simulink model "tasks500Hz"  (R2014a)
settings: Solver=FixedStepDiscrete  StartTime=0.0  StopTime=simTime  FixedStep=controlDT  RelTol=1e-3
values from neighbouring files (symbols this model uses):
  controlDT = 1 / 500    (= 0.002)    [setup.m]
  eepromConfig = p    [setup.m]
  triYawRateDenLP = p    [setup.m]
  triYawRateNumLP = p    [setup.m]
undefined symbols (not defined in the file or in its folder): DiscIntNeverNeededParam, mixHexX, mixQuadX, mixTri, mixY6
libraries: simulink x9, mahoneyAHRSlibrary x1
settings Model: Creator=John Ihlein  LastModifiedBy=John Ihlein
settings DataIOCC: SaveFormat=Structure  SaveOutput=off  SaveTime=off
settings OptimizationCC: InlineParams=on  DefaultUnderspecifiedDataType=single  InlineInvariantSignals=on  PassReuseOutputArgsAs=Individual arguments  StateBitsets=on  DataBitsets=on  ZeroExternalMemoryAtStartup=off  ZeroInternalMemoryAtStartup=off  EfficientFloat2IntCast=on  OptimizeModelRefInitCode=on  LifeSpan=1
settings DebuggingCC: ParameterPrecisionLossMsg=none  UniqueDataStoreMsg=error  AssertControl=DisableAll
settings HardwareCC: ProdLargestAtomicInteger=Integer  ProdLargestAtomicFloat=Float  ProdIntDivRoundTo=Zero  ProdEndianess=LittleEndian  ProdHWDeviceType=STMicroelectronics->STM32F4xx 32-bit Cortex-M4
settings RTWCC: SystemTargetFile=ert.tlc  GenCodeOnly=on  TemplateMakefile=ert_default_tmf  Description=Embedded Coder  ProcessScript=ert_make_rtw_hook
settings CodeAppCC: IgnoreCustomStorageClasses=off  IgnoreTestpoints=on
settings ERTTargetCC: ParMdlRefBuildCompliant=on  CompOptLevelCompliant=on  ConcurrentExecutionCompliant=on  IncludeMdlTerminateFcn=off  ERTFirstTimeCompliant=on  SupportNonFinite=off  ParenthesesLevel=Maximum  ModelStepFunctionPrototypeControlCompliant=on  CPPClassGenCompliant=on  InlinedParameterPlacement=Hierarchical  ERTCustomFileTemplate=example_file_process.tlc  ERTFilePackagingFormat=Compact

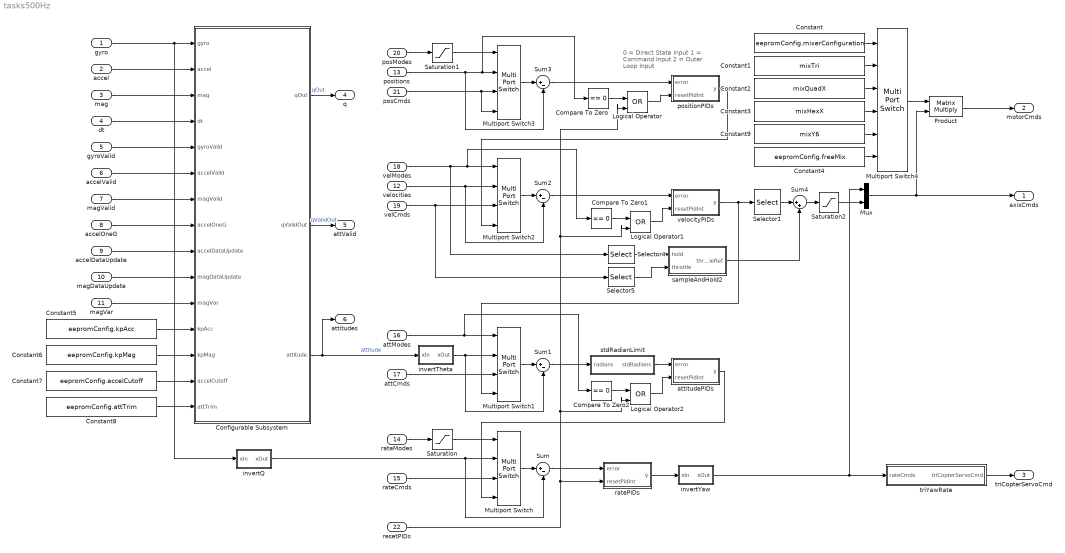
== system tasks500Hz ==
  note: 0 = Direct State Input
      | 1 = Command Input
      | 2 = Outer Loop Input
  "gyro " : Inport  OutDataTypeStr=single  PortDimensions=3  SampleTime=controlDT
  accel : Inport  Port=2  OutDataTypeStr=single  PortDimensions=3  SampleTime=controlDT
  mag : Inport  Port=3  OutDataTypeStr=single  PortDimensions=3  SampleTime=controlDT
  dt : Inport  Port=4  OutDataTypeStr=single  PortDimensions=1  SampleTime=controlDT
  gyroValid : Inport  Port=5  OutDataTypeStr=uint8  PortDimensions=1  SampleTime=controlDT
  accelValid : Inport  Port=6  OutDataTypeStr=uint8  PortDimensions=1  SampleTime=controlDT
  magValid : Inport  Port=7  OutDataTypeStr=uint8  PortDimensions=1  SampleTime=controlDT
  accelOneG : Inport  Port=8  OutDataTypeStr=single  PortDimensions=1  SampleTime=controlDT
  accelDataUpdate : Inport  Port=9  OutDataTypeStr=uint8  PortDimensions=1  SampleTime=controlDT
  magDataUpdate : Inport  Port=10  OutDataTypeStr=uint8  PortDimensions=1  SampleTime=controlDT
  magVar : Inport  Port=11  OutDataTypeStr=single  PortDimensions=1  SampleTime=controlDT
  velocities : Inport  Port=12  OutDataTypeStr=single  PortDimensions=3  SampleTime=controlDT
  positions : Inport  Port=13  OutDataTypeStr=single  PortDimensions=3  SampleTime=controlDT
  rateModes : Inport  Port=14  OutDataTypeStr=uint8  PortDimensions=3  SampleTime=controlDT
  rateCmds : Inport  Port=15  OutDataTypeStr=single  PortDimensions=3  SampleTime=controlDT
  attModes : Inport  Port=16  OutDataTypeStr=uint8  PortDimensions=3  SampleTime=controlDT
  attCmds : Inport  Port=17  OutDataTypeStr=single  PortDimensions=3  SampleTime=controlDT
  velModes : Inport  Port=18  OutDataTypeStr=uint8  PortDimensions=3  SampleTime=controlDT
  velCmds : Inport  Port=19  OutDataTypeStr=single  PortDimensions=3  SampleTime=controlDT
  posModes : Inport  Port=20  OutDataTypeStr=uint8  PortDimensions=3  SampleTime=controlDT
  posCmds : Inport  Port=21  OutDataTypeStr=single  PortDimensions=3  SampleTime=controlDT
  resetPIDs : Inport  Port=22  OutDataTypeStr=uint8  PortDimensions=1  SampleTime=controlDT
  Compare To Zero : simulink/Logic and Bit Operations/Compare To Zero  relop===  OutDataTypeStr=boolean
  Compare To Zero1 : simulink/Logic and Bit Operations/Compare To Zero  relop===  OutDataTypeStr=boolean
  Compare To Zero2 : simulink/Logic and Bit Operations/Compare To Zero  relop===  OutDataTypeStr=boolean
  Configurable Subsystem : Subsystem  BlockChoice=mahonyAHRS_MC
      settings: AttributesFormatString=%<BlockChoice>  MemberBlocks=mahonyAHRS_MC,mahonyAHRS_SL
      settings: TemplateBlock=|
      | mahoneyAHRSlibrary/Configurable
      | Subsystem
  Constant : Constant  Value=eepromConfig.mixerConfiguration  OutDataTypeStr=single  SampleTime=controlDT
  Constant1 : Constant  Value=mixTri  OutDataTypeStr=single  SampleTime=controlDT
  Constant2 : Constant  Value=mixQuadX  OutDataTypeStr=single  SampleTime=controlDT
  Constant3 : Constant  Value=mixHexX  OutDataTypeStr=single  SampleTime=controlDT
  Constant4 : Constant  Value=eepromConfig.freeMix  OutDataTypeStr=single  SampleTime=controlDT
  Constant5 : Constant  Value=eepromConfig.kpAcc  OutDataTypeStr=single  SampleTime=controlDT
  Constant6 : Constant  Value=eepromConfig.kpMag  OutDataTypeStr=single  SampleTime=controlDT
  Constant7 : Constant  Value=eepromConfig.accelCutoff  OutDataTypeStr=single  SampleTime=controlDT
  Constant8 : Constant  Value=eepromConfig.attTrim  OutDataTypeStr=single  SampleTime=controlDT
  Constant9 : Constant  Value=mixY6  OutDataTypeStr=single  SampleTime=controlDT
  Logical Operator : Logic  Operator=OR  IconShape=distinctive  AllPortsSameDT=off  OutDataTypeStr=boolean
  Logical Operator1 : Logic  Operator=OR  IconShape=distinctive  AllPortsSameDT=off  OutDataTypeStr=boolean
  Logical Operator2 : Logic  Operator=OR  IconShape=distinctive  AllPortsSameDT=off  OutDataTypeStr=boolean
  Multiport Switch4 : MultiPortSwitch  DataPortOrder=Zero-based contiguous  Inputs=5
  Multiport Switch{,1..3} (4 alike) : MultiPortSwitch  DataPortOrder=Zero-based contiguous
  Mux : Mux  Inputs=2
  Product : Product  Multiplication=Matrix(*)
  Saturation : Saturate  UpperLimit=2  LowerLimit=1
  Saturation1 : Saturate  UpperLimit=1  LowerLimit=0
  Saturation2 : Saturate  UpperLimit=4000  LowerLimit=2000
  Selector1 : Selector  IndexMode=Zero-based  InputPortWidth=3  Indices=[2]
  Selector4 : Selector  IndexMode=Zero-based  InputPortWidth=3  Indices=[2]
  Selector5 : Selector  IndexMode=Zero-based  InputPortWidth=3  Indices=[2]
  Sum{,1..3} (4 alike) : Sum  Inputs=|+-
  Sum4 : Sum  Inputs=|++
  attitudePIDs : Subsystem  mask{P=eepromConfig.attitudeP, I=eepromConfig.attitudeI, D=eepromConfig.attitudeD, N=100, Kb=100, pidLimit=eepromConfig.attitudeLimit}
      mask prompts: P "PID P Gain"; I "PID I Gain"; D "PID D Gain"; N "PID N"; Kb "PID Kb"; pidLimit "PID Limit"
  invertQ : Subsystem
  invertTheta : Subsystem
  invertYaw : Subsystem
  positionPIDs : Subsystem  mask{P=eepromConfig.positionP, I=eepromConfig.positionI, D=eepromConfig.positionD, N=100, Kb=100, pidLimit=eepromConfig.positionLimit}
      mask prompts: P "PID P Gain"; I "PID I Gain"; D "PID D Gain"; N "PID N"; Kb "PID Kb"; pidLimit "PID Limit"
  ratePIDs : Subsystem  mask{P=eepromConfig.rateP, I=eepromConfig.rateI, D=eepromConfig.rateD, N=100, Kb=100, pidLimit=eepromConfig.rateLimit}
      mask prompts: P "PID P Gain"; I "PID I Gain"; D "PID D Gain"; N "PID N"; Kb "PID Kb"; pidLimit "PID Limit"
  sampleAndHold2 : Subsystem
  stdRadianLimit : Subsystem
  triYawRate : Subsystem
  velocityPIDs : Subsystem  mask{P=eepromConfig.velocityP, I=eepromConfig.velocityI, D=eepromConfig.velocityD, N=100, Kb=100, pidLimit=eepromConfig.velocityLimit}
      mask prompts: P "PID P Gain"; I "PID I Gain"; D "PID D Gain"; N "PID N"; Kb "PID Kb"; pidLimit "PID Limit"
  axisCmds : Outport  OutDataTypeStr=single  PortDimensions=4  SampleTime=controlDT
  motorCmds : Outport  Port=2  OutDataTypeStr=single  PortDimensions=numMotors  SampleTime=controlDT
  triCopterServoCmd : Outport  Port=3  OutDataTypeStr=single  PortDimensions=1  SampleTime=controlDT
  q : Outport  Port=4  OutDataTypeStr=single  PortDimensions=[1 4]  SampleTime=controlDT
  attValid : Outport  Port=5  OutDataTypeStr=uint8  PortDimensions=1  SampleTime=controlDT
  attitudes : Outport  Port=6  OutDataTypeStr=single  PortDimensions=3  SampleTime=controlDT
  wires:
  attModes/1 -> Multiport Switch1/1, Compare To Zero2/1
  Sum1/1 -> stdRadianLimit/1(radians)
  velCmds/1 -> Multiport Switch2/3, Selector5/1
  velModes/1 -> Multiport Switch2/1, Compare To Zero1/1, Selector4/1
  Multiport Switch3/1 -> Sum3/1
  stdRadianLimit/1(stdRadians) -> attitudePIDs/1(error)
  attCmds/1 -> Multiport Switch1/3
  Multiport Switch/1 -> Sum/1
  Selector1/1 -> Sum4/1
  Multiport Switch2/1 -> Sum2/1
  velocityPIDs/1(y) -> Multiport Switch1/4, Selector1/1
  Sum3/1 -> positionPIDs/1(error)
  positions/1 -> Multiport Switch3/2, Compare To Zero/1, Sum3/2
  Multiport Switch1/1 -> Sum1/1
  Saturation/1 -> Multiport Switch/1
  sampleAndHold2/1(throttleRef) -> Sum4/2
  Selector4/1 -> sampleAndHold2/1(hold)
  Selector5/1 -> sampleAndHold2/2(throttle)
  rateModes/1 -> Saturation/1
  attitudePIDs/1(y) -> Multiport Switch/4
  posCmds/1 -> Multiport Switch3/3, Multiport Switch3/4
  rateCmds/1 -> Multiport Switch/3
  resetPIDs/1 -> Logical Operator/2, Logical Operator1/2, Logical Operator2/2, ratePIDs/2(resetPidInt)
  Sum/1 -> ratePIDs/1(error)
  velocities/1 -> Multiport Switch2/2, Sum2/2
  positionPIDs/1(y) -> Multiport Switch2/4
  Saturation1/1 -> Multiport Switch3/1
  posModes/1 -> Saturation1/1
  Mux/1 -> axisCmds/1, Product/2
  Sum4/1 -> Saturation2/1
  ratePIDs/1(y) -> invertYaw/1(xIn)
  Compare To Zero/1 -> Logical Operator/1
  Logical Operator/1 -> positionPIDs/2(resetPidInt)
  Compare To Zero1/1 -> Logical Operator1/1
  Logical Operator1/1 -> velocityPIDs/2(resetPidInt)
  Logical Operator2/1 -> attitudePIDs/2(resetPidInt)
  Compare To Zero2/1 -> Logical Operator2/1
  invertQ/1(xOut) -> Multiport Switch/2, Sum/2
  invertTheta/1(xOut) -> Multiport Switch1/2, Sum1/2
  Saturation2/1 -> Mux/2
  Constant/1 -> Multiport Switch4/1
  Constant1/1 -> Multiport Switch4/2
  Constant2/1 -> Multiport Switch4/3
  Constant3/1 -> Multiport Switch4/4
  Multiport Switch4/1 -> Product/1
  Product/1 -> motorCmds/1
  invertYaw/1(xOut) -> Mux/1, triYawRate/1(rateCmds)
  triYawRate/1(triCopterServoCmd) -> triCopterServoCmd/1
  Sum2/1 -> velocityPIDs/1(error)
  Configurable Subsystem/3(attitude) -> attitudes/1, invertTheta/1(xIn)  "attitude"
  Configurable Subsystem/2(qValidOut) -> attValid/1  "qValidOut"
  magDataUpdate/1 -> Configurable Subsystem/10(magDataUpdate)
  accel/1 -> Configurable Subsystem/2(accel)
  mag/1 -> Configurable Subsystem/3(mag)
  magValid/1 -> Configurable Subsystem/7(magValid)
  accelValid/1 -> Configurable Subsystem/6(accelValid)
  gyroValid/1 -> Configurable Subsystem/5(gyroValid)
  "gyro "/1 -> Configurable Subsystem/1(gyro), invertQ/1(xIn)
  Configurable Subsystem/1(qOut) -> q/1  "qOut"
  accelDataUpdate/1 -> Configurable Subsystem/9(accelDataUpdate)
  magVar/1 -> Configurable Subsystem/11(magVar)
  Constant5/1 -> Configurable Subsystem/12(kpAcc)
  Constant6/1 -> Configurable Subsystem/13(kpMag)
  Constant7/1 -> Configurable Subsystem/14(accelCutoff)
  Constant8/1 -> Configurable Subsystem/15(attTrim)
  dt/1 -> Configurable Subsystem/4(dt)
  accelOneG/1 -> Configurable Subsystem/8(accelOneG)
  Constant4/1 -> Multiport Switch4/6
  Constant9/1 -> Multiport Switch4/5

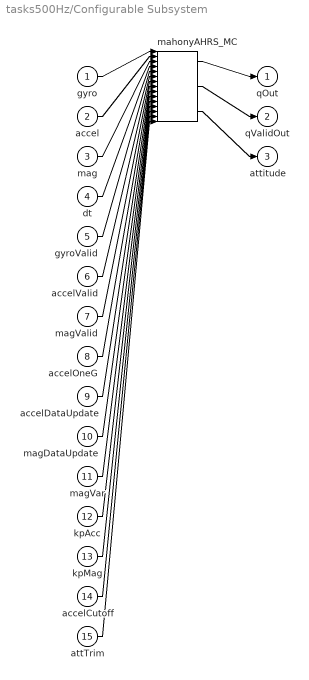
== system tasks500Hz/Configurable Subsystem ==
  gyro : Inport
  accel : Inport  Port=2
  mag : Inport  Port=3
  dt : Inport  Port=4
  gyroValid : Inport  Port=5
  accelValid : Inport  Port=6
  magValid : Inport  Port=7
  accelOneG : Inport  Port=8
  accelDataUpdate : Inport  Port=9
  magDataUpdate : Inport  Port=10
  magVar : Inport  Port=11
  kpAcc : Inport  Port=12
  kpMag : Inport  Port=13
  accelCutoff : Inport  Port=14
  attTrim : Inport  Port=15
  mahonyAHRS_MC : mahoneyAHRSlibrary/mahonyAHRS_MC
  qOut : Outport
  qValidOut : Outport  Port=2
  attitude : Outport  Port=3
  wires:
  gyro/1 -> mahonyAHRS_MC/1
  accel/1 -> mahonyAHRS_MC/2
  mag/1 -> mahonyAHRS_MC/3
  dt/1 -> mahonyAHRS_MC/4
  gyroValid/1 -> mahonyAHRS_MC/5
  accelValid/1 -> mahonyAHRS_MC/6
  magValid/1 -> mahonyAHRS_MC/7
  accelOneG/1 -> mahonyAHRS_MC/8
  accelDataUpdate/1 -> mahonyAHRS_MC/9
  magDataUpdate/1 -> mahonyAHRS_MC/10
  magVar/1 -> mahonyAHRS_MC/11
  kpAcc/1 -> mahonyAHRS_MC/12
  kpMag/1 -> mahonyAHRS_MC/13
  accelCutoff/1 -> mahonyAHRS_MC/14
  attTrim/1 -> mahonyAHRS_MC/15
  mahonyAHRS_MC/1 -> qOut/1
  mahonyAHRS_MC/2 -> qValidOut/1
  mahonyAHRS_MC/3 -> attitude/1

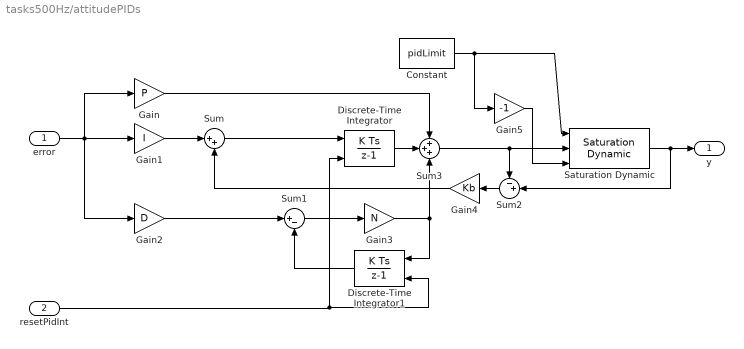
== system tasks500Hz/attitudePIDs ==
  error : Inport
  resetPidInt : Inport  Port=2
  Constant : Constant  Value=pidLimit
  Discrete-Time Integrator : DiscreteIntegrator  ExternalReset=level  SampleTime=-1  ICPrevOutput=DiscIntNeverNeededParam  ICPrevScaledInput=DiscIntNeverNeededParam
  Discrete-Time Integrator1 : DiscreteIntegrator  ExternalReset=level  SampleTime=-1  ICPrevOutput=DiscIntNeverNeededParam  ICPrevScaledInput=DiscIntNeverNeededParam
  Gain : Gain  Gain=P
  Gain1 : Gain  Gain=I
  Gain2 : Gain  Gain=D
  Gain3 : Gain  Gain=N
  Gain4 : Gain  Gain=Kb
  Gain5 : Gain  Gain=-1
  Saturation Dynamic : simulink/Discontinuities/Saturation Dynamic  OutMin=[]  OutMax=[]  OutDataTypeStr=Inherit: Same as second input  OutDataType=fixdt(1, 16)  OutScaling=2^-10  DoSatur=off
  Sum : Sum  Inputs=|++
  Sum1 : Sum  Inputs=|+-
  Sum2 : Sum  Inputs=-+|
  Sum3 : Sum  Inputs=+++
  y : Outport
  wires:
  Constant/1 -> Saturation Dynamic/1, Gain5/1
  Gain5/1 -> Saturation Dynamic/3
  Gain/1 -> Sum3/1
  error/1 -> Gain1/1, Gain2/1, Gain/1
  Saturation Dynamic/1 -> Sum2/2, y/1
  Discrete-Time Integrator1/1 -> Sum1/2
  Sum2/1 -> Gain4/1
  Discrete-Time Integrator/1 -> Sum3/2
  Gain2/1 -> Sum1/1
  Gain3/1 -> Sum3/3, Discrete-Time Integrator1/1
  Sum/1 -> Discrete-Time Integrator/1
  Gain1/1 -> Sum/1
  Sum3/1 -> Sum2/1, Saturation Dynamic/2
  Sum1/1 -> Gain3/1
  Gain4/1 -> Sum/2
  resetPidInt/1 -> Discrete-Time Integrator/2, Discrete-Time Integrator1/2

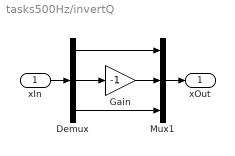
== system tasks500Hz/invertQ ==
  xIn : Inport
  Demux : Demux  Outputs=3
  Gain : Gain  Gain=-1
  Mux1 : Mux  Inputs=3
  xOut : Outport
  wires:
  Gain/1 -> Mux1/2
  Demux/3 -> Mux1/3
  Demux/1 -> Mux1/1
  Mux1/1 -> xOut/1
  Demux/2 -> Gain/1
  xIn/1 -> Demux/1

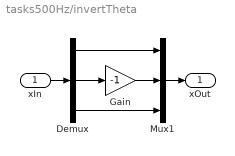
== system tasks500Hz/invertTheta ==
  xIn : Inport
  Demux : Demux  Outputs=3
  Gain : Gain  Gain=-1
  Mux1 : Mux  Inputs=3
  xOut : Outport
  wires:
  Demux/3 -> Mux1/3
  Demux/1 -> Mux1/1
  xIn/1 -> Demux/1
  Demux/2 -> Gain/1
  Mux1/1 -> xOut/1
  Gain/1 -> Mux1/2

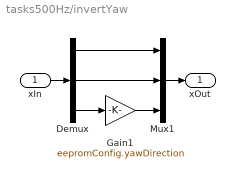
== system tasks500Hz/invertYaw ==
  xIn : Inport
  Demux : Demux  Outputs=3
  Gain1 : Gain  Gain=eepromConfig.yawDirection
  Mux1 : Mux  Inputs=3
  xOut : Outport
  wires:
  Gain1/1 -> Mux1/3
  Demux/2 -> Mux1/2
  Mux1/1 -> xOut/1
  xIn/1 -> Demux/1
  Demux/1 -> Mux1/1
  Demux/3 -> Gain1/1

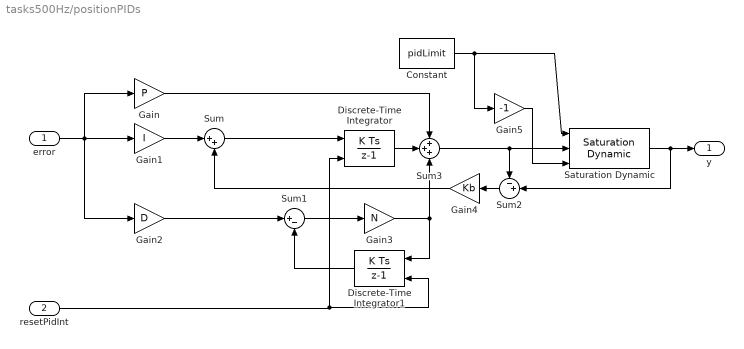
== system tasks500Hz/positionPIDs ==
  error : Inport
  resetPidInt : Inport  Port=2
  Constant : Constant  Value=pidLimit
  Discrete-Time Integrator : DiscreteIntegrator  ExternalReset=level  SampleTime=-1  ICPrevOutput=DiscIntNeverNeededParam  ICPrevScaledInput=DiscIntNeverNeededParam
  Discrete-Time Integrator1 : DiscreteIntegrator  ExternalReset=level  SampleTime=-1  ICPrevOutput=DiscIntNeverNeededParam  ICPrevScaledInput=DiscIntNeverNeededParam
  Gain : Gain  Gain=P
  Gain1 : Gain  Gain=I
  Gain2 : Gain  Gain=D
  Gain3 : Gain  Gain=N
  Gain4 : Gain  Gain=Kb
  Gain5 : Gain  Gain=-1
  Saturation Dynamic : simulink/Discontinuities/Saturation Dynamic  OutMin=[]  OutMax=[]  OutDataTypeStr=Inherit: Same as second input  OutDataType=fixdt(1, 16)  OutScaling=2^-10  DoSatur=off
  Sum : Sum  Inputs=|++
  Sum1 : Sum  Inputs=|+-
  Sum2 : Sum  Inputs=-+|
  Sum3 : Sum  Inputs=+++
  y : Outport
  wires:
  Constant/1 -> Saturation Dynamic/1, Gain5/1
  Gain5/1 -> Saturation Dynamic/3
  Gain/1 -> Sum3/1
  error/1 -> Gain1/1, Gain2/1, Gain/1
  Saturation Dynamic/1 -> Sum2/2, y/1
  Discrete-Time Integrator1/1 -> Sum1/2
  Sum2/1 -> Gain4/1
  Discrete-Time Integrator/1 -> Sum3/2
  Gain2/1 -> Sum1/1
  Gain3/1 -> Sum3/3, Discrete-Time Integrator1/1
  Sum/1 -> Discrete-Time Integrator/1
  Gain1/1 -> Sum/1
  Sum3/1 -> Sum2/1, Saturation Dynamic/2
  Sum1/1 -> Gain3/1
  Gain4/1 -> Sum/2
  resetPidInt/1 -> Discrete-Time Integrator/2, Discrete-Time Integrator1/2

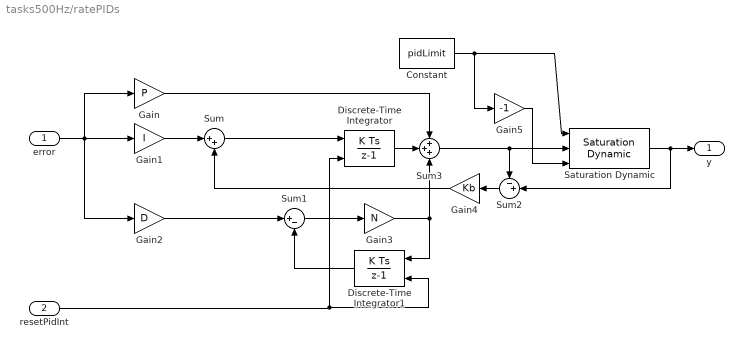
== system tasks500Hz/ratePIDs ==
  error : Inport
  resetPidInt : Inport  Port=2
  Constant : Constant  Value=pidLimit
  Discrete-Time Integrator : DiscreteIntegrator  ExternalReset=level  SampleTime=-1  ICPrevOutput=DiscIntNeverNeededParam  ICPrevScaledInput=DiscIntNeverNeededParam
  Discrete-Time Integrator1 : DiscreteIntegrator  ExternalReset=level  SampleTime=-1  ICPrevOutput=DiscIntNeverNeededParam  ICPrevScaledInput=DiscIntNeverNeededParam
  Gain : Gain  Gain=P
  Gain1 : Gain  Gain=I
  Gain2 : Gain  Gain=D
  Gain3 : Gain  Gain=N
  Gain4 : Gain  Gain=Kb
  Gain5 : Gain  Gain=-1
  Saturation Dynamic : simulink/Discontinuities/Saturation Dynamic  OutMin=[]  OutMax=[]  OutDataTypeStr=Inherit: Same as second input  OutDataType=fixdt(1, 16)  OutScaling=2^-10  DoSatur=off
  Sum : Sum  Inputs=|++
  Sum1 : Sum  Inputs=|+-
  Sum2 : Sum  Inputs=-+|
  Sum3 : Sum  Inputs=+++
  y : Outport
  wires:
  resetPidInt/1 -> Discrete-Time Integrator1/2, Discrete-Time Integrator/2
  Gain4/1 -> Sum/2
  Sum1/1 -> Gain3/1
  Sum3/1 -> Saturation Dynamic/2, Sum2/1
  Gain1/1 -> Sum/1
  Sum/1 -> Discrete-Time Integrator/1
  Gain3/1 -> Discrete-Time Integrator1/1, Sum3/3
  Gain2/1 -> Sum1/1
  Discrete-Time Integrator/1 -> Sum3/2
  Sum2/1 -> Gain4/1
  Discrete-Time Integrator1/1 -> Sum1/2
  Saturation Dynamic/1 -> y/1, Sum2/2
  error/1 -> Gain/1, Gain2/1, Gain1/1
  Gain/1 -> Sum3/1
  Gain5/1 -> Saturation Dynamic/3
  Constant/1 -> Gain5/1, Saturation Dynamic/1

== system tasks500Hz/sampleAndHold2 ==
  hold : Inport
  throttle : Inport  Port=2
  Unit Delay : UnitDelay  SampleTime=-1
  u2~=0 : Switch  Criteria=u2 ~= 0
  throttleRef : Outport
  wires:
  throttle/1 -> u2~=0/3
  hold/1 -> u2~=0/2
  u2~=0/1 -> throttleRef/1, Unit Delay/1
  Unit Delay/1 -> u2~=0/1

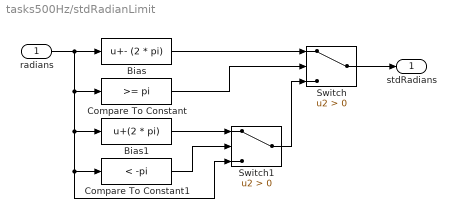
== system tasks500Hz/stdRadianLimit ==
  radians : Inport
  Bias : Bias  Bias=- (2 * pi)
  Bias1 : Bias  Bias=(2 * pi)
  Compare To Constant : simulink/Logic and Bit Operations/Compare To Constant  relop=>=  const=pi  OutDataTypeStr=boolean
  Compare To Constant1 : simulink/Logic and Bit Operations/Compare To Constant  relop=<  const=-pi  OutDataTypeStr=boolean
  Switch : Switch  Criteria=u2 > Threshold
  Switch1 : Switch  Criteria=u2 > Threshold
  stdRadians : Outport
  wires:
  Switch/1 -> stdRadians/1
  radians/1 -> Bias/1, Compare To Constant/1, Bias1/1, Compare To Constant1/1, Switch1/3
  Switch1/1 -> Switch/3
  Compare To Constant1/1 -> Switch1/2
  Bias1/1 -> Switch1/1
  Bias/1 -> Switch/1
  Compare To Constant/1 -> Switch/2

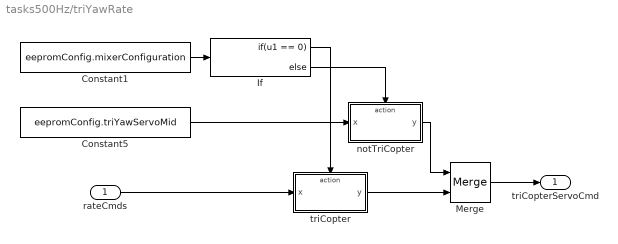
== system tasks500Hz/triYawRate ==
  rateCmds : Inport
  Constant1 : Constant  Value=eepromConfig.mixerConfiguration  SampleTime=controlDT
  Constant5 : Constant  Value=eepromConfig.triYawServoMid  SampleTime=controlDT
  If : If  IfExpression=u1 == 0
  Merge : Merge
  notTriCopter : Subsystem  TreatAsAtomicUnit=on
  triCopter : Subsystem  TreatAsAtomicUnit=on
  triCopterServoCmd : Outport
  wires:
  Constant1/1 -> If/1
  rateCmds/1 -> triCopter/1(x)
  If/1 -> triCopter/Action
  If/2 -> notTriCopter/Action
  Constant5/1 -> notTriCopter/1(x)
  Merge/1 -> triCopterServoCmd/1
  triCopter/1(y) -> Merge/2
  notTriCopter/1(y) -> Merge/1

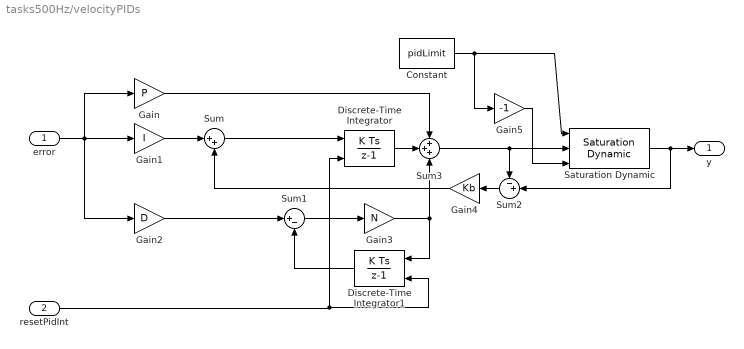
== system tasks500Hz/velocityPIDs ==
  error : Inport
  resetPidInt : Inport  Port=2
  Constant : Constant  Value=pidLimit
  Discrete-Time Integrator : DiscreteIntegrator  ExternalReset=level  SampleTime=-1  ICPrevOutput=DiscIntNeverNeededParam  ICPrevScaledInput=DiscIntNeverNeededParam
  Discrete-Time Integrator1 : DiscreteIntegrator  ExternalReset=level  SampleTime=-1  ICPrevOutput=DiscIntNeverNeededParam  ICPrevScaledInput=DiscIntNeverNeededParam
  Gain : Gain  Gain=P
  Gain1 : Gain  Gain=I
  Gain2 : Gain  Gain=D
  Gain3 : Gain  Gain=N
  Gain4 : Gain  Gain=Kb
  Gain5 : Gain  Gain=-1
  Saturation Dynamic : simulink/Discontinuities/Saturation Dynamic  OutMin=[]  OutMax=[]  OutDataTypeStr=Inherit: Same as second input  OutDataType=fixdt(1, 16)  OutScaling=2^-10  DoSatur=off
  Sum : Sum  Inputs=|++
  Sum1 : Sum  Inputs=|+-
  Sum2 : Sum  Inputs=-+|
  Sum3 : Sum  Inputs=+++
  y : Outport
  wires:
  resetPidInt/1 -> Discrete-Time Integrator1/2, Discrete-Time Integrator/2
  Gain4/1 -> Sum/2
  Sum1/1 -> Gain3/1
  Sum3/1 -> Saturation Dynamic/2, Sum2/1
  Gain1/1 -> Sum/1
  Sum/1 -> Discrete-Time Integrator/1
  Gain3/1 -> Discrete-Time Integrator1/1, Sum3/3
  Gain2/1 -> Sum1/1
  Discrete-Time Integrator/1 -> Sum3/2
  Sum2/1 -> Gain4/1
  Discrete-Time Integrator1/1 -> Sum1/2
  Saturation Dynamic/1 -> y/1, Sum2/2
  error/1 -> Gain/1, Gain2/1, Gain1/1
  Gain/1 -> Sum3/1
  Gain5/1 -> Saturation Dynamic/3
  Constant/1 -> Gain5/1, Saturation Dynamic/1

== system tasks500Hz/triYawRate/notTriCopter ==
  x : Inport
  Action Port : ActionPort  ActionType=else
  y : Outport
  wires:
  x/1 -> y/1

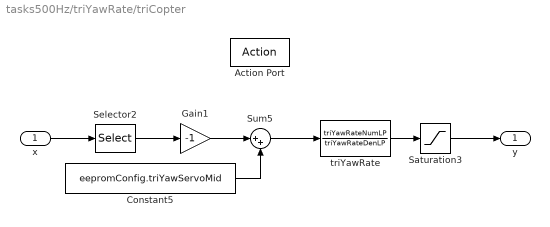
== system tasks500Hz/triYawRate/triCopter ==
  x : Inport
  Action Port : ActionPort  ActionType=then
  Constant5 : Constant  Value=eepromConfig.triYawServoMid  SampleTime=controlDT
  Gain1 : Gain  Gain=-1
  Saturation3 : Saturate  UpperLimit=eepromConfig.triYawServoMax  LowerLimit=eepromConfig.triYawServoMin
  Selector2 : Selector  IndexMode=Zero-based  InputPortWidth=3  Indices=[2]
  Sum5 : Sum  Inputs=|++
  triYawRate : DiscreteTransferFcn  Numerator=triYawRateNumLP  Denominator=triYawRateDenLP  SampleTime=controlDT
  y : Outport
  wires:
  Gain1/1 -> Sum5/1
  Sum5/1 -> triYawRate/1
  Constant5/1 -> Sum5/2
  Selector2/1 -> Gain1/1
  triYawRate/1 -> Saturation3/1
  x/1 -> Selector2/1
  Saturation3/1 -> y/1
